simulink model "phan1_bai2b_kieu1_2016"  (R2016a)
settings: Solver=VariableStepAuto  SolverMode=SingleTasking  StartTime=0.0  StopTime=30  RelTol=1e-3
libraries: simulink x1
settings Model: Creator=inhuo  LastModifiedBy=inhuo
settings DataIOCC: ReturnWorkspaceOutputs=on
settings DebuggingCC: SFUnexpectedBacktrackingDiag=error  SFNoUnconditionalDefaultTransitionDiag=error
settings SFSimCC: SimUseLocalCustomCode=on
settings RTWCC: RTWUseLocalCustomCode=on
settings GRTTargetCC: TargetLangStandard=C99 (ISO)  GeneratePreprocessorConditionals=Use local settings
settings ConfigComp: CovMetricSettings=dwe  CovHtmlReporting=off  CovSaveCumulativeToWorkspaceVar=off  CovSaveSingleToWorkspaceVar=off  CovExternalEMLEnable=on

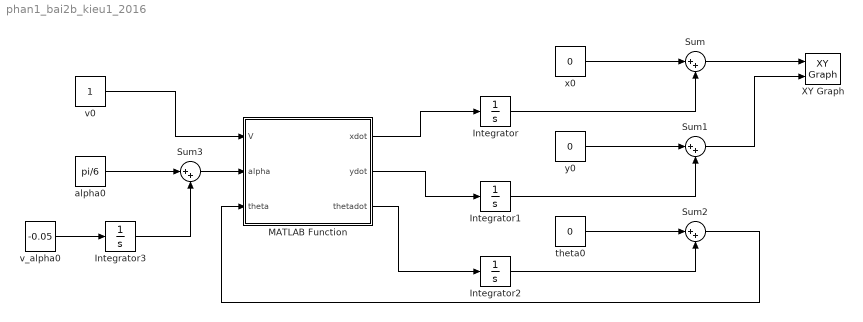
== system phan1_bai2b_kieu1_2016 ==
  Integrator{,1..3} (4 alike) : Integrator
  MATLAB Function : MATLAB Function  TreatAsAtomicUnit=on
  Sum{,1..3} (4 alike) : Sum  Inputs=|++
  XY Graph : simulink/Sinks/XY Graph  xmin=-20  xmax=20  ymin=-20  ymax=20  st=-1
  alpha0 : Constant  Value=pi/6
  theta0 : Constant  Value=0
  v0 : Constant
  v_alpha0 : Constant  Value=-0.05
  x0 : Constant  Value=0
  y0 : Constant  Value=0
  wires:
  Sum1/1 -> XY Graph/2
  MATLAB Function/3(thetadot) -> Integrator2/1
  MATLAB Function/2(ydot) -> Integrator1/1
  Sum2/1 -> MATLAB Function/3(theta)
  Sum/1 -> XY Graph/1
  x0/1 -> Sum/1
  Integrator2/1 -> Sum2/2
  Integrator1/1 -> Sum1/2
  theta0/1 -> Sum2/1
  MATLAB Function/1(xdot) -> Integrator/1
  y0/1 -> Sum1/1
  Integrator/1 -> Sum/2
  alpha0/1 -> Sum3/1
  v0/1 -> MATLAB Function/1(V)
  v_alpha0/1 -> Integrator3/1
  Integrator3/1 -> Sum3/2
  Sum3/1 -> MATLAB Function/2(alpha)

== matlab function phan1_bai2b_kieu1_2016/MATLAB Function ==
  data: V input; xdot output; alpha input; theta input; ydot output; thetadot output
function [xdot , ydot , thetadot]= fcn(V,alpha,theta)

    d = sqrt (2.5 + 0.1 * 9);

    if abs(alpha) > pi/4
        alpha = pi/4*sign(alpha);
    end

    if V > (1.5 + 0.03 * 9) %lon hon van toc cuc dai
        V = (1.5 + 0.03 * 9)
    end
    % case 1:
    xdot = V*cos(alpha)*cos(theta);
    ydot = V*cos(alpha)*sin(theta);
    thetadot =V*sin(alpha)/d;
end

% case 1 
% xdot = V*cos(alpha)*cos(theta);
% ydot = V*cos(alpha)*sin(theta);
% thetadot =V*sin(alpha)/d;

% case 2
% xdot = V*cos(theta);
% ydot = V*sin(theta);
% thetadot =V*tan(alpha)/d;
